simulink model "perturb_and_observe_MPPT"  (R2023a)
settings: Solver=VariableStepAuto  StartTime=0.0  StopTime=10.0  RelTol=1e-3
settings Model: Creator=rahul  LastModifiedBy=rahul

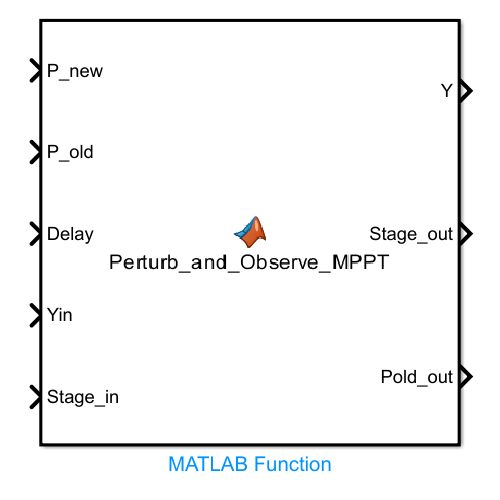
[thumbnail: Simulink's stored preview of the top-level diagram]
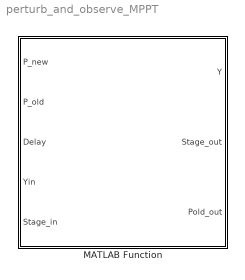
== system perturb_and_observe_MPPT ==
  MATLAB Function : MATLAB Function  TreatAsAtomicUnit=on

== matlab function perturb_and_observe_MPPT/MATLAB Function ==
  data: P_new input; Y output; P_old input; Delay input; Yin input; Stage_in input; Stage_out output; Pold_out output
function [Y,Stage_out,Pold_out]=Perturb_and_Observe_MPPT(P_new,P_old,Delay,Yin,Stage_in) 
c=0.05;
Pold_out=P_old;
Y=Yin;
Stage_out= Stage_in;
if Delay == 0

    if Stage_in==0
                    if  P_new>P_old
                    Y=Yin+c;
                    Pold_out=P_new;
                    elseif P_new<P_old
                    Y=Yin-c;
                    Stage_out=1;
                    Pold_out=P_new;
                    end
                    Pold_out=P_new;
   end
    
   if Stage_in==1
                    if P_new>P_old
                    Y=Yin-c;
                     Pold_out=P_new;
                    elseif P_new<P_old
                    Y=Yin+c;
                    Stage_out=0;
                    Pold_out=P_new;
                    end
                    Pold_out=P_new;
   end           
end
